simulink model "Child"  (R2023a)
settings: Solver=FixedStepAuto  StartTime=0.0  StopTime=inf  RelTol=1e-3
libraries: androiduilib x6, androidcommunicationlib x5, androidsensorlib x3, androidaudiovideolib x3
settings Model: Creator=tamiz  LastModifiedBy=srira
settings OptimizationCC: EnhancedBackFolding=on  PassReuseOutputArgsAs=Individual arguments  ZeroExternalMemoryAtStartup=off  ZeroInternalMemoryAtStartup=off  MaxStackSize=64  OptimizeBlockOrder=speed  DifferentSizesBufferReuse=on  UseRowMajorAlgorithm=on  OptimizationCustomize=off  EfficientTunableParamExpr=on
settings DebuggingCC: ParameterTunabilityLossMsg=error
settings HardwareCC: ProdBitPerPointer=32  ProdBitPerSizeT=32  ProdBitPerPtrDiffT=32  ProdLargestAtomicInteger=Long  ProdLargestAtomicFloat=Double  ProdWordSize=32  ProdHWDeviceType=ARM Compatible->ARM Cortex  UseEmbeddedCoderFeatures=off  UseSimulinkCoderFeatures=off
settings RTWCC: Description=Embedded Coder  SystemTargetFile=ert.tlc  HardwareBoard=Android Device  TLCOptions="-aInlineSetEventsForThisBaseRateFcn=TLC_FALSE -aSuppressMultiTaskScheduler=TLC_FALSE  -aRateBasedStepFcn=0"  TemplateMakefile=ert_default_tmf  RTWVerbose=off  Toolchain=Android SDK/NDK Tools
settings CodeAppCC: ForceParamTrailComments=on  IgnoreCustomStorageClasses=off  OperatorAnnotations=on  SimulinkDataObjDesc=on  SFDataObjDesc=on  InsertBlockDesc=on
settings ERTTargetCC: SupportNonInlinedSFcns=on

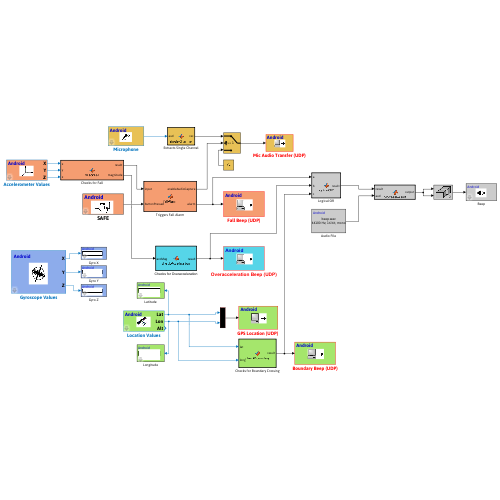
[thumbnail: Simulink's stored preview of the top-level diagram]
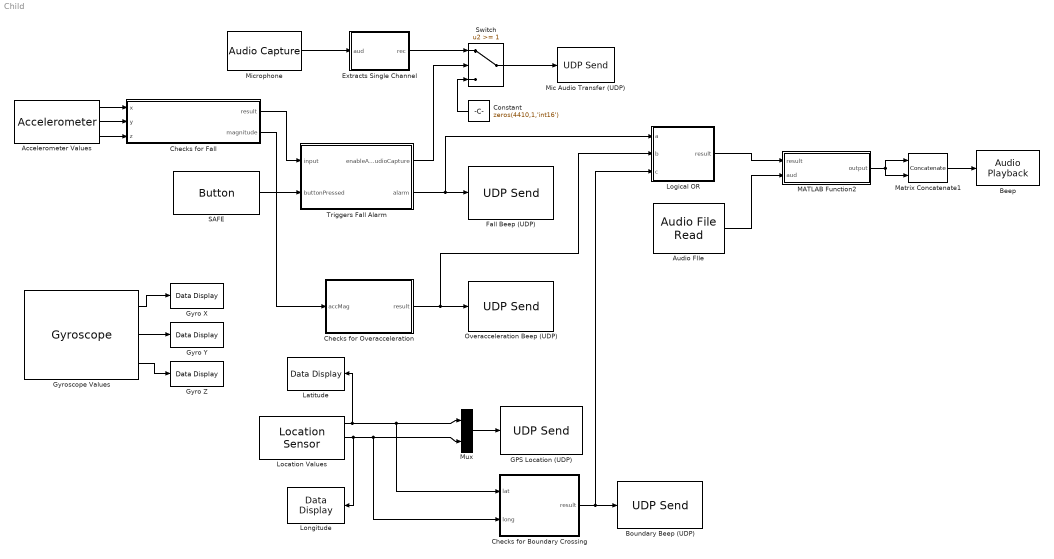
== system Child ==
  " SAFE " : androiduilib/Button  ButtonState=Not pressed  ButtonId=Child/_SAFE_  State=off  SampleTime=0.1  BlockPlatform=Android
  Accelerometer Values : androidsensorlib/Accelerometer  OutputVector=off  SampleTime=0.1  BlockPlatform=Android
  Audio FIle : androidaudiovideolib/Audio File Read  FileName=E:\IITGN\Child_Safety\beep.wav  FrameSize=4410
  Beep : androidaudiovideolib/Audio Playback  SampleFreq=44100  AudioSamplingFreq=44100  SampleTime=0.1  DeviceStr=0  QueueDuration=0  BlockPlatform=Android
  Boundary Beep (UDP) : androidcommunicationlib/UDP Send  remoteURL='10.7.13.55'  remotePort=25002  localURL='0.0.0.0'  localPortSource=Automatically determine  localPort=-1  sampletime=-1  blockPlatform=Android  separateLengthPort=0
  Checks for Boundary Crossing : MATLAB Function  TreatAsAtomicUnit=on
  Checks for Fall : MATLAB Function  TreatAsAtomicUnit=on
  Checks for Overacceleration : MATLAB Function  TreatAsAtomicUnit=on
  Constant : Constant  Value=zeros(4410,1,'int16')  VectorParams1D=off
  Extracts Single Channel : MATLAB Function  TreatAsAtomicUnit=on
  Fall Beep (UDP) : androidcommunicationlib/UDP Send  remoteURL='10.7.13.55'  remotePort=25001  localURL='0.0.0.0'  localPortSource=Automatically determine  localPort=-1  sampletime=-1  blockPlatform=Android  separateLengthPort=0
  "GPS Location (UDP) " : androidcommunicationlib/UDP Send  remoteURL='10.7.13.55'  remotePort=25000  localURL='0.0.0.0'  localPortSource=Automatically determine  localPort=-1  sampletime=-1  blockPlatform=Android  separateLengthPort=0
  Gyro X : androiduilib/Data Display  DataDisplayId=Child/Gyro_X  Format=Float  Precision=6  SimulateUsing=Code generation  blockPlatform=Android
  Gyro Y : androiduilib/Data Display  DataDisplayId=Child/Gyro_Y  Format=Float  Precision=6  SimulateUsing=Code generation  blockPlatform=Android
  Gyro Z : androiduilib/Data Display  DataDisplayId=Child/Gyro_Z  Format=Float  Precision=6  SimulateUsing=Code generation  blockPlatform=Android
  Gyroscope Values : androidsensorlib/Gyroscope  OutputVector=off  SampleTime=0.1  BlockPlatform=Android
  Latitude : androiduilib/Data Display  DataDisplayId=Child/Latitude  Format=Float  Precision=10  SimulateUsing=Code generation  blockPlatform=Android
  Location Values : androidsensorlib/Location Sensor  OutputVector=off  SampleTime=0.1  BlockPlatform=Android
  Logical OR : MATLAB Function  TreatAsAtomicUnit=on
  Longitude : androiduilib/Data Display  DataDisplayId=Child/Longitude  Format=Float  Precision=10  SimulateUsing=Code generation  blockPlatform=Android
  MATLAB Function2 : MATLAB Function  TreatAsAtomicUnit=on
  Matrix Concatenate1 : Concatenate  Mode=Multidimensional array  ConcatenateDimension=2
  Mic Audio Transfer (UDP) : androidcommunicationlib/UDP Send  remoteURL='10.7.13.55'  remotePort=25004  localURL='0.0.0.0'  localPortSource=Automatically determine  localPort=-1  sampletime=-1  blockPlatform=Android  separateLengthPort=0
  Microphone : androidaudiovideolib/Audio Capture  SampleFreq=44100  FrameSize=4410  SampleTime=0.1  SimulateUsing=Code generation  DeviceStr=0  QueueDuration=0  BlockPlatform=Android  AudioSamplingFreq=44100
  Mux : Mux  Inputs=2
  Overacceleration Beep (UDP) : androidcommunicationlib/UDP Send  remoteURL='10.7.13.55'  remotePort=25003  localURL='0.0.0.0'  localPortSource=Automatically determine  localPort=-1  sampletime=-1  blockPlatform=Android  separateLengthPort=0
  Switch : Switch  Threshold=1  SaturateOnIntegerOverflow=off  InputSameDT=off
  Triggers Fall Alarm : MATLAB Function  TreatAsAtomicUnit=on
  wires:
  Audio FIle/1 -> MATLAB Function2/2(aud)
  Location Values/1 -> Checks for Boundary Crossing/1(lat), Mux/1, Latitude/1
  Location Values/2 -> Longitude/1, Checks for Boundary Crossing/2(long), Mux/2
  Accelerometer Values/1 -> Checks for Fall/1(x)
  Accelerometer Values/2 -> Checks for Fall/2(y)
  Accelerometer Values/3 -> Checks for Fall/3(z)
  Gyroscope Values/1 -> Gyro X/1
  Gyroscope Values/2 -> Gyro Y/1
  Gyroscope Values/3 -> Gyro Z/1
  Matrix Concatenate1/1 -> Beep/1
  MATLAB Function2/1(output) -> Matrix Concatenate1/2, Matrix Concatenate1/1
  Mux/1 -> "GPS Location (UDP) "/1
  Checks for Boundary Crossing/1(result) -> Logical OR/3(c), Boundary Beep (UDP)/1
  Logical OR/1(result) -> MATLAB Function2/1(result)
  " SAFE "/1 -> Triggers Fall Alarm/2(buttonPressed)
  Checks for Fall/1(result) -> Triggers Fall Alarm/1(input)
  Triggers Fall Alarm/2(alarm) -> Logical OR/1(a), Fall Beep (UDP)/1
  Triggers Fall Alarm/1(enableAudioCapture) -> Switch/2
  Switch/1 -> Mic Audio Transfer (UDP)/1
  Constant/1 -> Switch/3
  Microphone/1 -> Extracts Single Channel/1(aud)
  Extracts Single Channel/1(rec) -> Switch/1
  Checks for Fall/2(magnitude) -> Checks for Overacceleration/1(accMag)
  Checks for Overacceleration/1(result) -> Overacceleration Beep (UDP)/1, Logical OR/2(b)

== matlab function Child/Checks for Fall ==
  data: x input; result output; y input; z input; magnitude output
function [result, magnitude] = checkFall(x, y, z)
    % Calculate the magnitude of acceleration
    magnitude = sqrt(x^2 + y^2 + z^2);
    acceleration_break_point = 60;
    % Check if magnitude is greater than or equal to 15
    if magnitude >= acceleration_break_point
        result = true;
    else
        result = false;
    end
end

== matlab function Child/Checks for Boundary Crossing ==
  data: lat input; result output; long input
function result = checkBoundary(lat, long)
    prec = 10;
    LAT_HOME= 23.2099905000*(10^prec);
    LONG_HOME = 72.6837888000*(10^prec);
    LAT_PC = 23.210634*(10^prec);
    LONG_PC = 72.684499*(10^prec);
    
    D = ((LAT_PC - LAT_HOME)^2 + (LONG_PC- LONG_HOME)^2)^(0.5); % safe distance
    d = ((LAT_HOME - lat*(10^prec))^2+(LONG_HOME - long*(10^prec))^2)^(0.5); % actual distance
    
    if d >= D
        result = true;
    else
        result = false;
    end
end
% 23.210706431153127
% 72.68441190143524

== matlab function Child/MATLAB Function2 ==
  data: result input; output output; aud input
function output = processResult(result, aud)
    if result == 1
        output = aud;
    else
        output = zeros(4410,1,'int16');
    end
end

== matlab function Child/Logical OR ==
  data: a input; result output; b input; c input
function result = logicalOR(a, b, c)
    % Logical OR function
    result = a || b || c;
end

== matlab function Child/Triggers Fall Alarm ==
  data: enableAudioCapture output; input input; alarm output; buttonPressed input
function [enableAudioCapture, alarm] = fallAlarm(input, buttonPressed)
    persistent timerStarted;
    persistent danger;
    
    enableAudioCapture = 0;
    alarm = false;
    
    if isempty(danger)
        danger = 0;
    end

    if input == 1
        danger = 1;
        if isempty(timerStarted)
            timerStarted = true; 
            tic; % Start the timer
        end

        if timerStarted == false
            timerStarted = true; 
            tic; % Start the timer
        end
    end

    if danger == 1
        alarm = true;
        if toc >= 5 && buttonPressed ~= 1
            enableAudioCapture = 1;
        elseif buttonPressed == 1
            timerStarted = false;
            danger = 0;
            alarm = false; 
        end
    end
end

== matlab function Child/Extracts Single Channel ==
  data: aud input; rec output
function rec = singleChannel(aud)
    rec = aud(:,2);

== matlab function Child/Checks for Overacceleration ==
  data: accMag input; result output
function result = checkAcceleration(accMag)
    % Check if the acceleration magnitude is greater than 25
    if accMag > 25
        result = true; 
    else
        result = false; 
    end
end
